simulink model "velocityramp"  (R2021a)
settings: Solver=FixedStepAuto  StartTime=0.0  StopTime=inf  FixedStep=0.02  RelTol=1e-3
libraries: robotlib x3
settings Model: EnablePacing=on  Creator=safwan  LastModifiedBy=sprinkle
settings OptimizationCC: EnhancedBackFolding=on  PassReuseOutputArgsAs=Individual arguments  ZeroExternalMemoryAtStartup=off  ZeroInternalMemoryAtStartup=off  MaxStackSize=64  OptimizeBlockOrder=speed  DifferentSizesBufferReuse=on  EfficientTunableParamExpr=on
settings DebuggingCC: ParameterTunabilityLossMsg=error
settings HardwareCC: ProdBitPerPointer=32  ProdBitPerSizeT=32  ProdBitPerPtrDiffT=32  ProdLargestAtomicFloat=None  ProdIntDivRoundTo=Undefined  ProdEndianess=Unspecified  ProdWordSize=32  ProdHWDeviceType=Generic->Unspecified (assume 32-bit Generic)
settings SFSimCC: MATLABDynamicMemAlloc=off
settings RTWCC: SystemTargetFile=ert.tlc  HardwareBoard=Robot Operating System (ROS)  TLCOptions="-aInlineSetEventsForThisBaseRateFcn=TLC_FALSE -aSuppressMultiTaskScheduler=TLC_FALSE  -aRateBasedStepFcn=0"  TemplateMakefile=ert_default_tmf  Toolchain=Catkin  TargetLang=C++
settings CodeAppCC: ForceParamTrailComments=on  IgnoreCustomStorageClasses=off  OperatorAnnotations=on  SimulinkDataObjDesc=on  SFDataObjDesc=on  InsertBlockDesc=on
settings ERTTargetCC: SupportContinuousTime=on

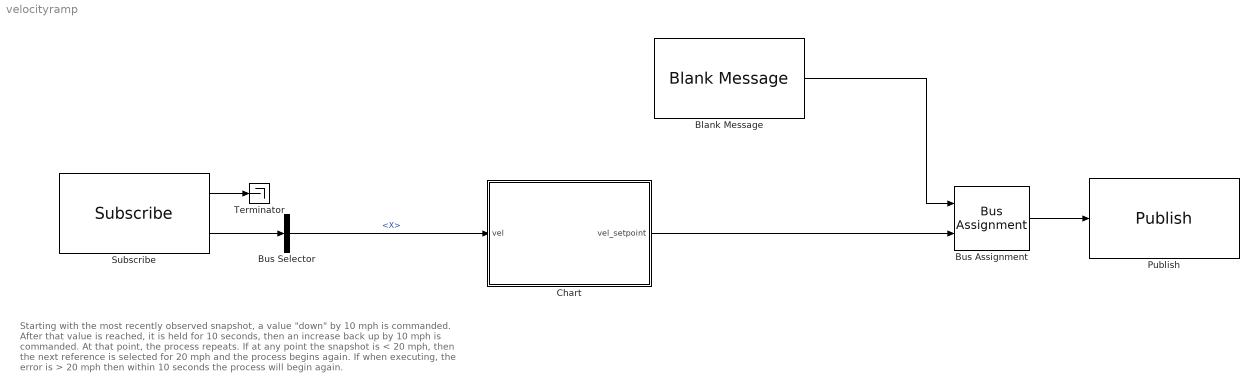
== system velocityramp ==
  note: Starting with the most recently observed snapshot, a value "down" by 10 mph is
      | commanded. After that value is reached, it is held for 10 seconds, then an increase back up by 10 mph is commanded.
      |
      | At that point, the process repeats.
      |
      | If at any point the snapshot is < 20 mph, then the next reference is selected for 20 mph and the process begins again.
      |
      | If when executing, the error is > 20 mph then within 10 seconds the process will begin again.
  Blank Message : robotlib/Blank Message  messageClass=Message  entityType=geometry_msgs/Twist  messageType=geometry_msgs/Twist  SampleTime=-1  legacyBusStruct=off
  Bus Assignment : BusAssignment  AssignedSignals=Linear.X
  Bus Selector : BusSelector  OutputSignals=Linear.X
  Chart : Stateflow chart  TreatAsAtomicUnit=on
  Publish : robotlib/Publish  topicSource=Specify your own  topic=vel_setpoint  messageType=geometry_msgs/Twist  legacyBusStruct=off  messageQueueLength=1
  Subscribe : robotlib/Subscribe  topicSource=Specify your own  topic=vel  messageType=geometry_msgs/Twist  SampleTime=-1  legacyBusStruct=off  messageQueueLength=1
  Terminator : Terminator
  wires:
  Blank Message/1 -> Bus Assignment/1
  Bus Assignment/1 -> Publish/1
  Subscribe/1 -> Terminator/1
  Subscribe/2 -> Bus Selector/1
  Bus Selector/1 -> Chart/1(vel)  "<X>"
  Chart/1(vel_setpoint) -> Bus Assignment/2

== stateflow chart velocityramp/Chart ==
  state reset
    entry: vel_setpoint = max(vel,15);
  state HoldAtPeak1
  state RaiseBy10
    entry: vel_setpoint=vel_setpoint + 5;
  state HoldAtPeak
  state HoldAtValley
  state DropBy10
    entry: vel_setpoint = vel_setpoint - 5;
  (default) -> reset
  HoldAtPeak1 -> reset [order 2] : [abs(vel - vel_setpoint) > 10]
  HoldAtPeak1 -> reset [order 1] : after(10,sec)
  RaiseBy10 -> reset [order 2] : [abs(vel-vel_setpoint) > 10]
  RaiseBy10 -> HoldAtPeak1 [order 1] : [abs(vel - vel_setpoint) < 0.1]
  HoldAtValley -> reset [order 2] : [abs(vel-vel_setpoint) > 10]
  DropBy10 -> reset [order 2] : [abs(vel-vel_setpoint) > 10]
  reset -> HoldAtPeak
  HoldAtPeak -> reset [order 2] : [abs(vel - vel_setpoint) > 10]
  HoldAtValley -> RaiseBy10 [order 1] : after(10,sec)
  HoldAtPeak -> DropBy10 [order 1] : after(10,sec)
  DropBy10 -> HoldAtValley [order 1] : [abs(vel - vel_setpoint) < 0.1]
  data: vel input; vel_setpoint output
